simulink model "danhgia_chatluong_chuabutre"  (R2020a)
settings: Solver=ode1be  StartTime=0.0  StopTime=Tmophong  FixedStep=Ts  RelTol=1e-3
values from neighbouring files (symbols this model uses):
  L = 30e-3    (= 0.03)    [init.m]    (also in init_khongbutre.m)
  omega_Ref = 2*pi*50    (= 314.159265359)    [init.m]    (also in init_khongbutre.m)
  R = 6    [init.m]    (also in init_khongbutre.m; kalmanfilter1.m = 4)
  Ts = 50e-6    (= 5e-05)    [init.m]    (also in init_khongbutre.m)
libraries: nesl_utility x18, ee_lib x17, fl_lib x4
settings Model: Creator=tinh  LastModifiedBy=Tinh_deptrai
settings SolverCC: NumberNewtonIterations=3
settings DataIOCC: ExternalInput=sinA,sinB,sinC  LoadExternalInput=on
settings SimscapeCC: SimscapeLogToSDI=on

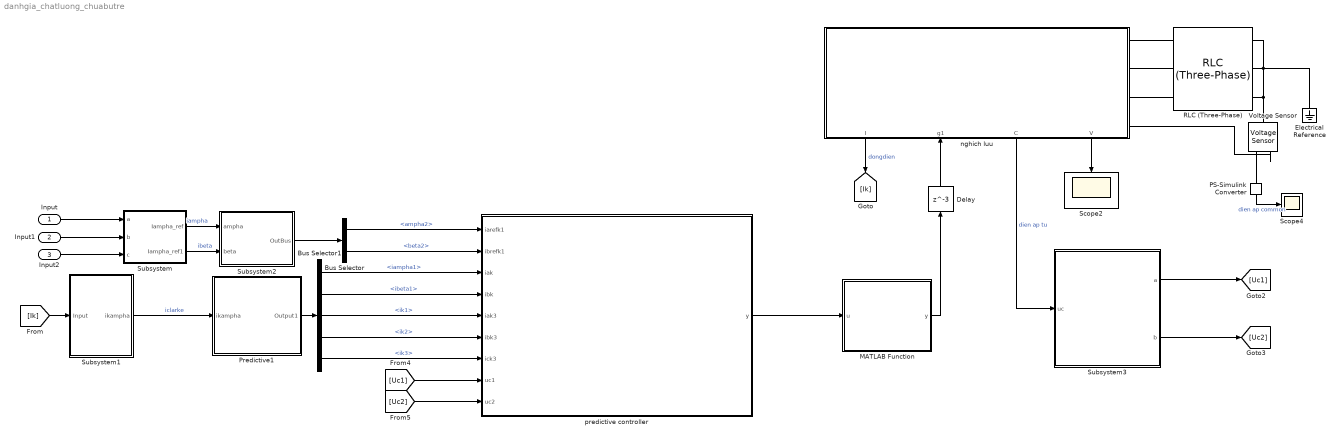
== system danhgia_chatluong_chuabutre ==
  Input : Inport
  Input1 : Inport  Port=2
  Input2 : Inport  Port=3
  Bus Selector : BusSelector  OutputSignals=ampha2,beta2
  Bus Selector1 : BusSelector  OutputSignals=iampha1,ibeta1,ik1,ik2,ik3
  Delay : Delay  DelayLength=3
  Electrical Reference : fl_lib/Electrical/Electrical Elements/Electrical Reference
  MATLAB Function : MATLAB Function  TreatAsAtomicUnit=on
  PS-Simulink Converter : nesl_utility/PS-Simulink Converter  PhysicalDomain=network_engine_domain  SubClassName=ps_output  LeftPortType=input  RightPortType=output  PseudoPeriodic=off  Frequencies=[]  Unit=inherit  AffineConversion=off
  Predictive1 : Subsystem
  RLC (Three-Phase) : ee_lib/Passive/RLC Assemblies/RLC (Three-Phase)  component_structure=4  R=R Ohm  L=L H  IL0=[0, 0, 0] A  C=1e-6 F  VC0=[0, 0, 0] V  R_parasitic=1e-6 Ohm  G_parasitic=1e-6 1/Ohm
      settings: SourceProductBaseCode=PS  InternalSimscapePortConfiguration="{\"Bottom\":[],\"Left\":[{\"id\":\"a1\",\"label\":\"a1\",\"type\":\"foundation.electrical.electrical\"},{\"id\":\"b1\",\"label\":\"b1\",\"type\":\"foundation.electrical.electrical\"},{\"id\":\"c1\",\"label\":\"c1\",\"type\":\"foundation.electrical.electrical\"}],\"Right\":[{\"id\":\"a2\",\"label\":\"a2\",\"type\":\"foundation.electrical.electrical\"},{\"id\":\"b2\",\"label\":\"b2\",\"type\":\"foundation.electrical.electrical\"},{\"id\":\"c2\",\"label\":\"c2\",\"type\":\"foundation.electrical.electrical\"}],\"Top\":[]}"
  Scope2 : Scope
  Scope4 : Scope
  Subsystem : Subsystem
  Subsystem1 : Subsystem
  Subsystem2 : Subsystem
  Subsystem3 : Subsystem
  Voltage Sensor : fl_lib/Electrical/Electrical Sensors/Voltage Sensor
  nghich luu : Subsystem
      settings: PortSchema="{\"entries\":[{\"content\":{\"sides\":[{\"content\":{\"connectorIds\":[]},\"type\":\"ConnectorPlacement.EquallySpacedRectSide\",\"uuid\":\"1f21bf9d-b3c4-4ef8-831a-50a976b6aa65\"},{\"content\":{\"connectorIds\":[\"RConn1\",\"RConn2\",\"RConn3\",\"RConn4\"],\"side\":\"RIGHT\"},\"type\":\"ConnectorPlacement.EquallySpacedRectSide\",\"uuid\":\"0787168a-1f3c-4831-aef7-a1860c607723\"},{\"content\":{\"connectorIds\":[],\"side\":\"TOP\"},\"type\":\"ConnectorPlacement.EquallySpacedRectSide\",\"uuid\":\"c9cfdced-0897-45ca-aa61-726ea781df92\"},{\"content\":{\"connectorIds\":[\"Out1\",\"In1\",\"Out2\",\"Out3\"],\"side\":\"BOTTOM\"},\"type\":\"ConnectorPlacement.EquallySpacedRectSide\",\"uuid\":\"0f797b02-a78f-4846-a0f4-57f75c54f7ea\"}]},\"type\":\"ConnectorPlacement.EquallySpacedConnector\",\"uuid\":\"5e077d9d-cbda-4f20-95e3-2cacb065a3ee\"}],\"packageUris\":[\"http://schema.mathworks.com/mf0/Connector/19700101\"],\"version\":\"1.0\"}"
  predictive controller : MATLAB Function  TreatAsAtomicUnit=on
  wires:
  Input2/1 -> Subsystem/3(c)
  Subsystem/1(Iampha_ref) -> Subsystem2/1(ampha)  "iampha"
  Subsystem/2(Iampha_ref1) -> Subsystem2/2(beta)  "ibeta"
  Input/1 -> Subsystem/1(a)
  Input1/1 -> Subsystem/2(b)
  MATLAB Function/1(y) -> Delay/1
  Delay/1 -> nghich luu/1(g1)
  nghich luu/2(C) -> Subsystem3/1(uc)  "dien ap tu"
  nghich luu/3(V) -> Scope2/1
  nghich luu/1(I) -> [Ik]  "dongdien"
  Bus Selector/1 -> predictive controller/1(iarefk1)  "<ampha2>"
  Bus Selector/2 -> predictive controller/2(ibrefk1)  "<beta2>"
  Subsystem2/1(OutBus) -> Bus Selector/1
  Bus Selector1/1 -> predictive controller/3(iak)  "<iampha1>"
  Bus Selector1/2 -> predictive controller/4(ibk)  "<ibeta1>"
  Bus Selector1/3 -> predictive controller/5(iak3)  "<ik1>"
  Bus Selector1/4 -> predictive controller/6(ibk3)  "<ik2>"
  Bus Selector1/5 -> predictive controller/7(ick3)  "<ik3>"
  Subsystem3/1(a) -> [Uc1]
  Subsystem3/2(b) -> [Uc2]
  PS-Simulink Converter/1 -> Scope4/1  "dien ap common"
  Predictive1/1(Output1) -> Bus Selector1/1
  [Ik] -> Subsystem1/1(Input)
  Subsystem1/1(ikampha) -> Predictive1/1(ikampha)  "iclarke"
  [Uc1] -> predictive controller/8(uc1)
  [Uc2] -> predictive controller/9(uc2)
  predictive controller/1(y) -> MATLAB Function/1(u)
  connections:
  RLC (Three-Phase)/RConn3 -- RLC (Three-Phase)/RConn2 -- RLC (Three-Phase)/RConn1 -- Electrical Reference/LConn1 -- Voltage Sensor/LConn1
  RLC (Three-Phase)/LConn1 -- nghich luu/RConn1
  RLC (Three-Phase)/LConn2 -- nghich luu/RConn2
  RLC (Three-Phase)/LConn3 -- nghich luu/RConn3
  Voltage Sensor/RConn2 -- nghich luu/RConn4
  PS-Simulink Converter/LConn1 -- Voltage Sensor/RConn1

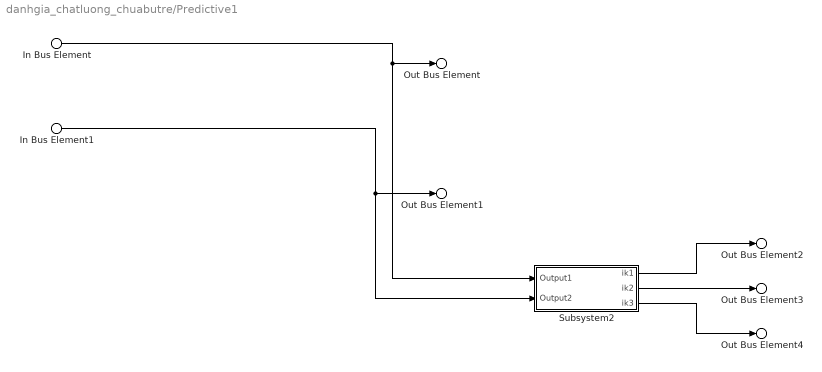
== system danhgia_chatluong_chuabutre/Predictive1 ==
  In Bus Element : Inport  PortName=ikampha  Element=Iampha
  In Bus Element1 : Inport  PortName=ikampha  Element=Ibeta
  Subsystem2 : Subsystem
  Out Bus Element : Outport  PortName=Output1  Element=iampha1
  Out Bus Element1 : Outport  PortName=Output1  Element=ibeta1
  Out Bus Element2 : Outport  PortName=Output1  Element=ik1
  Out Bus Element3 : Outport  PortName=Output1  Element=ik2
  Out Bus Element4 : Outport  PortName=Output1  Element=ik3
  wires:
  In Bus Element/1 -> Out Bus Element/1, Subsystem2/1(Output1)
  In Bus Element1/1 -> Out Bus Element1/1, Subsystem2/2(Output2)
  Subsystem2/1(ik1) -> Out Bus Element2/1
  Subsystem2/2(ik2) -> Out Bus Element3/1
  Subsystem2/3(ik3) -> Out Bus Element4/1

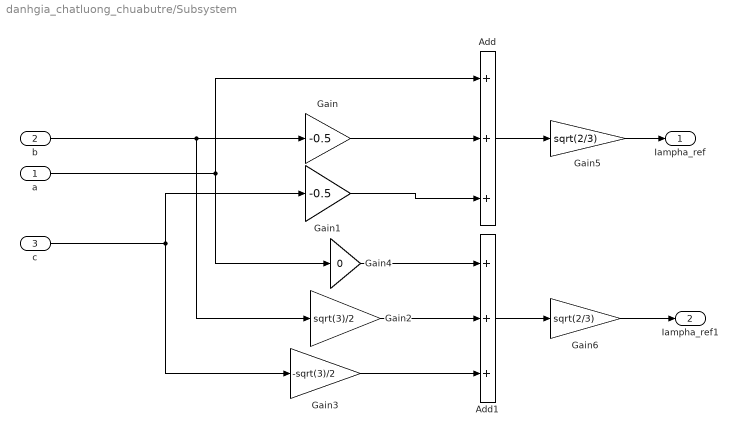
== system danhgia_chatluong_chuabutre/Subsystem ==
  a : Inport
  b : Inport  Port=2
  c : Inport  Port=3
  Add : Sum  Inputs=+++
  Add1 : Sum  Inputs=+++
  Gain : Gain  Gain=-0.5
  Gain1 : Gain  Gain=-0.5
  Gain2 : Gain  Gain=sqrt(3)/2
  Gain3 : Gain  Gain=-sqrt(3)/2
  Gain4 : Gain  Gain=0
  Gain5 : Gain  Gain=sqrt(2/3)
  Gain6 : Gain  Gain=sqrt(2/3)
  Iampha_ref : Outport
  Iampha_ref1 : Outport  Port=2
  wires:
  Add1/1 -> Gain6/1
  Gain3/1 -> Add1/3
  Gain2/1 -> Add1/2
  Gain1/1 -> Add/3
  c/1 -> Gain3/1, Gain1/1
  Gain/1 -> Add/2
  b/1 -> Gain2/1, Gain/1
  Add/1 -> Gain5/1
  a/1 -> Add/1, Gain4/1
  Gain4/1 -> Add1/1
  Gain5/1 -> Iampha_ref/1
  Gain6/1 -> Iampha_ref1/1

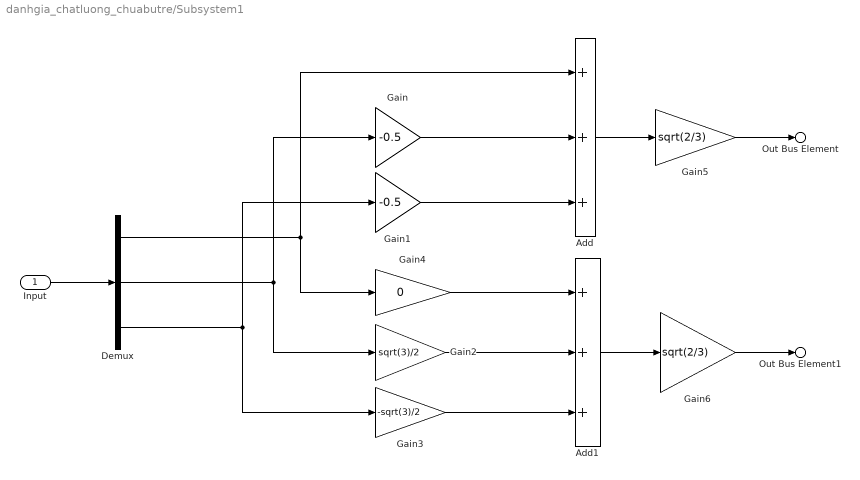
== system danhgia_chatluong_chuabutre/Subsystem1 ==
  Input : Inport
  Add : Sum  Inputs=+++
  Add1 : Sum  Inputs=+++
  Demux : Demux  Outputs=3
  Gain : Gain  Gain=-0.5
  Gain1 : Gain  Gain=-0.5
  Gain2 : Gain  Gain=sqrt(3)/2
  Gain3 : Gain  Gain=-sqrt(3)/2
  Gain4 : Gain  Gain=0
  Gain5 : Gain  Gain=sqrt(2/3)
  Gain6 : Gain  Gain=sqrt(2/3)
  Out Bus Element : Outport  PortName=ikampha  Element=Iampha
  Out Bus Element1 : Outport  PortName=ikampha  Element=Ibeta
  wires:
  Add1/1 -> Gain6/1
  Gain3/1 -> Add1/3
  Gain2/1 -> Add1/2
  Gain1/1 -> Add/3
  Demux/3 -> Gain3/1, Gain1/1
  Gain/1 -> Add/2
  Demux/2 -> Gain2/1, Gain/1
  Add/1 -> Gain5/1
  Demux/1 -> Add/1, Gain4/1
  Gain4/1 -> Add1/1
  Gain5/1 -> Out Bus Element/1
  Gain6/1 -> Out Bus Element1/1
  Input/1 -> Demux/1

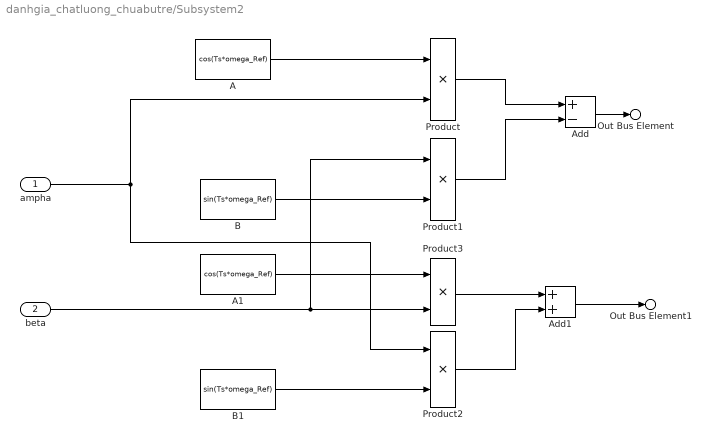
== system danhgia_chatluong_chuabutre/Subsystem2 ==
  ampha : Inport
  beta : Inport  Port=2
  A : Constant  Value=cos(Ts*omega_Ref)
  A1 : Constant  Value=cos(Ts*omega_Ref)
  Add : Sum  Inputs=+-
  Add1 : Sum
  B : Constant  Value=sin(Ts*omega_Ref)
  B1 : Constant  Value=sin(Ts*omega_Ref)
  Product{,1..3} (4 alike) : Product
  Out Bus Element : Outport  PortName=OutBus  Element=ampha2
  Out Bus Element1 : Outport  PortName=OutBus  Element=beta2
  wires:
  A/1 -> Product/1
  B/1 -> Product1/2
  ampha/1 -> Product2/1, Product/2
  beta/1 -> Product1/1, Product3/2
  A1/1 -> Product3/1
  B1/1 -> Product2/2
  Product/1 -> Add/1
  Product1/1 -> Add/2
  Product3/1 -> Add1/1
  Product2/1 -> Add1/2
  Add/1 -> Out Bus Element/1
  Add1/1 -> Out Bus Element1/1

== system danhgia_chatluong_chuabutre/Subsystem3 ==
  uc : Inport
  Demux1 : Demux  Outputs=2
  a : Outport
  b : Outport  Port=2
  wires:
  uc/1 -> Demux1/1
  Demux1/1 -> a/1
  Demux1/2 -> b/1

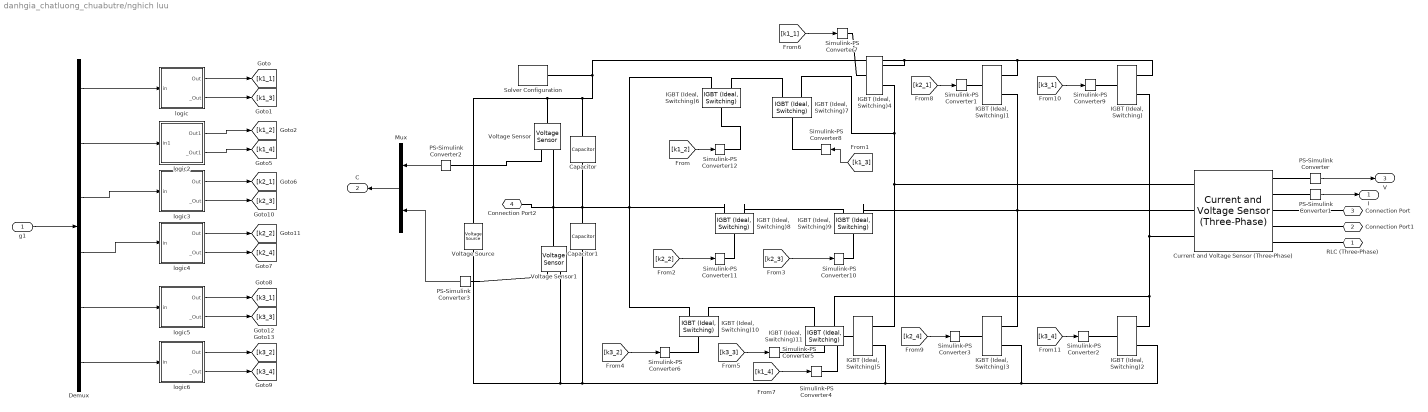
== system danhgia_chatluong_chuabutre/nghich luu ==
  g1 : Inport
  Capacitor : ee_lib/Passive/Capacitor  cap_option=0  c=0.0022 F  Cvec=[1e-05, 1e-06] F  Vvec=[0, 10] V  CV_table_symmetry=1  f_vec=[1, 10] kHz  DFext_vec=[.8, 1.2]  C_tol=5  enable_C_tol=0  tol_distribution=1  nSigma=4  r=1e-6 Ohm  g=0 1/Ohm  averaging_period=0 s  enable_operating_limits=1  operating_limit_action=2  max_working_voltage_range=[30, 60] V  power_rating=200 W  enable_faults=0  fault_action=1  Cscale_faulted=100  R_faulted=1e-3 Ohm  G_faulted=0 1/Ohm  tau_fault=1e-3 s  enable_temporal_fault=0  t_fault=1 s  enable_behavioral_fault=0  max_permissible_voltage_range=[-100, 100] V  t_fail_on_voltage=1 s  i_specify=off  i_priority=None  i=0 A  i_nominal_specify=off  i_nominal_unit=A  i_nominal_value=1  v_specify=on  v_priority=High  v=50 V  v_nominal_specify=off  v_nominal_unit=V  v_nominal_value=1  vc_specify=on  vc_priority=High  vc=50 V  vc_nominal_specify=off  vc_nominal_unit=V  vc_nominal_value=1
  Capacitor1 : ee_lib/Passive/Capacitor  cap_option=0  c=0.0022 F  Cvec=[1e-05, 1e-06] F  Vvec=[0, 10] V  CV_table_symmetry=1  f_vec=[1, 10] kHz  DFext_vec=[.8, 1.2]  C_tol=5  enable_C_tol=0  tol_distribution=1  nSigma=4  r=1e-6 Ohm  g=0 1/Ohm  averaging_period=0 s  enable_operating_limits=1  operating_limit_action=2  max_working_voltage_range=[30, 60] V  power_rating=200 W  enable_faults=0  fault_action=1  Cscale_faulted=100  R_faulted=1e-3 Ohm  G_faulted=0 1/Ohm  tau_fault=1e-3 s  enable_temporal_fault=0  t_fault=1 s  enable_behavioral_fault=0  max_permissible_voltage_range=[-100, 100] V  t_fail_on_voltage=1 s  i_specify=off  i_priority=None  i=0 A  i_nominal_specify=off  i_nominal_unit=A  i_nominal_value=1  v_specify=on  v_priority=High  v=50 V  v_nominal_specify=off  v_nominal_unit=V  v_nominal_value=1  vc_specify=on  vc_priority=High  vc=50 V  vc_nominal_specify=off  vc_nominal_unit=V  vc_nominal_value=1
  Current and Voltage Sensor (Three-Phase) : ee_lib/Sensors & Transducers/Current and Voltage Sensor (Three-Phase)  vMeasurementType=ee.enum.vmeasurement.lg  outputUnit=ee.enum.unit.si  SRated=100e6 V*A  VRated=24e3 V  I_specify=off  I_priority=None  I=[ 0 0 0 ] A  I_nominal_specify=off  I_nominal_unit=A  I_nominal_value=1  V_specify=off  V_priority=None  V=[ 0 0 0 ] V  V_nominal_specify=off  V_nominal_unit=V  V_nominal_value=1
      settings: SourceProductBaseCode=PS  InternalSimscapePortConfiguration="{\"Bottom\":[],\"Left\":[{\"id\":\"a1\",\"label\":\"a1\",\"type\":\"foundation.electrical.electrical\"},{\"id\":\"b1\",\"label\":\"b1\",\"type\":\"foundation.electrical.electrical\"},{\"id\":\"c1\",\"label\":\"c1\",\"type\":\"foundation.electrical.electrical\"}],\"Right\":[{\"id\":\"V_output\",\"label\":\"V\",\"type\":\"output\"},{\"id\":\"I_output\",\"label\":\"I\",\"type\":\"output\"},{\"id\":\"a2\",\"label\":\"a2\",\"type\":\"foundation.electrical.electrical\"},{\"id\":\"b2\",\"label\":\"b2\",\"type\":\"foundation.electrical.electrical\"},{\"id\":\"c2\",\"label\":\"c2\",\"type\":\"foundation.electrical.electrical\"}],\"Top\":[]}"
  Demux : Demux  Outputs=6
  IGBT (Ideal, Switching){,1..11} (12 alike) : ee_lib/Semiconductors & Converters/IGBT (Ideal, Switching)  Vf=0.8 V  Ron=0.001 Ohm  Goff=1e-6 1/Ohm  Vth=0.5 V  diode_param=2  diode_Vf=0.8 V  diode_Ron=0.001 Ohm  diode_Goff=1e-6 1/Ohm  diode_C=50e-9 F  diode_iRM=-235 A  diode_iF=300 A  diode_idot=-50 A/us  diode_trr_param=1  diode_trr_factor=3  diode_trr=15 us  diode_Qrr=1500 s*uA  thermal_loss_option=2  Voff=300 V  Tau=1e-4 s  Tj=[298.15, 398.15] K  Iout_scalar=600 A  Eon_scalar=22.86e-3 J  Eoff_scalar=17.14e-3 J  Von_scalar=2.7 V  Iout_data=[0, 10, 50, 100, 200, 400, 600] A  Eon_data=[0, .29, 1.43, 2.86, 5.71, 13.14, 22.86; 0, .57, 2.63, 5.14, 10.29, 20.57, 30.29] * 1e-3 J  Eoff_data=[0, .21, 1.07, 2.14, 4.29, 9.86, 17.14; 0, .43, 1.97, 3.86, 7.71, 15.43, 22.71] * 1e-3 J  Von_data=[0, 1.1, 1.3, 1.45, 1.75, 2.25, 2.7; 0, 1, 1.15, 1.35, 1.7, 2.35, 3] V
  Mux : Mux  Inputs=2
  PS-Simulink Converter : nesl_utility/PS-Simulink Converter  PhysicalDomain=network_engine_domain  SubClassName=ps_output  LeftPortType=input  RightPortType=output  PseudoPeriodic=off  Frequencies=[]  Unit=inherit  AffineConversion=off
  PS-Simulink Converter1 : nesl_utility/PS-Simulink Converter  PhysicalDomain=network_engine_domain  SubClassName=ps_output  LeftPortType=input  RightPortType=output  PseudoPeriodic=off  Frequencies=[]  Unit=inherit  AffineConversion=off
  PS-Simulink Converter2 : nesl_utility/PS-Simulink Converter  PhysicalDomain=network_engine_domain  SubClassName=ps_output  LeftPortType=input  RightPortType=output  PseudoPeriodic=off  Frequencies=[]  Unit=V  AffineConversion=off
  PS-Simulink Converter3 : nesl_utility/PS-Simulink Converter  PhysicalDomain=network_engine_domain  SubClassName=ps_output  LeftPortType=input  RightPortType=output  PseudoPeriodic=off  Frequencies=[]  Unit=V  AffineConversion=off
  Simulink-PS Converter{1..12} (12 alike) : nesl_utility/Simulink-PS Converter  PhysicalDomain=network_engine_domain  SubClassName=ps_input  LeftPortType=input  RightPortType=output  PseudoPeriodic=off  Frequencies=[]  NoiseDistribution=none  NoiseParameters=[]  Unit=V  AffineConversion=off  FilteringAndDerivatives=provide  SimscapeFilterOrder=1  InputFilterTimeConstant=0.001  UdotUserProvided=0
  Solver Configuration : nesl_utility/Solver Configuration  PhysicalDomain=network_engine_domain  SubClassName=solver  LeftPortType=input  RightPortType=generic  Tones=[]  Harmonics=[]  SimulateNoise=off  Profile=off  UseLocalSampling=off  EnableSwitchedLinearOptims=on  FrequencyDomain=off  UseCCode=off  RelTol=0.001  AbsTol=1e-06  MinStep=1e-09  ToWorkspace=off  RevertToSquareIcSolve=off  NumHomotopyIterations=100  PhasorMode=off  PhasorModeNumHarmonics=1  DoDC=off  ResidualTolerance=10e-06  UseLocalSolver=on  LocalSolverChoice=NE_TRAPEZOIDAL_ADVANCER  LocalSolverSampleTime=Ts  DoFixedCost=off  MaxNonlinIter=3  MaxModeIter=2  LinearAlgebra=auto  EquationFormulation=NE_TIME_EF  DelaysMemoryBudget=1024  AutomaticFiltering=on  FilteringTimeConstant=0.001  PartitionStorageMethod=AS_NEEDED  PartitionMemoryBudget=1024  PartitionMethod=ROBUST
  Voltage Sensor : fl_lib/Electrical/Electrical Sensors/Voltage Sensor
  Voltage Sensor1 : fl_lib/Electrical/Electrical Sensors/Voltage Sensor
  Voltage Source : ee_lib/Sources/Voltage Source  dc_voltage=Vdc V  ac_voltage=0 V  ac_shift=0 rad  ac_frequency=0 Hz  noise_mode=0  PSD=0 V^2/Hz  repeatability=1  auto_seed=418932850  user_seed=0  sample_time=1e-3 s  i_specify=off  i_priority=None  i=0 A  i_nominal_specify=off  i_nominal_unit=A  i_nominal_value=1  v_specify=off  v_priority=None  v=0 V  v_nominal_specify=off  v_nominal_unit=V  v_nominal_value=1
  logic : Subsystem
  logic2 : Subsystem
  logic3 : Subsystem
  logic4 : Subsystem
  logic5 : Subsystem
  logic6 : Subsystem
  RLC (Three-Phase) : PMIOPort  Side=Right
  Connection Port1 : PMIOPort  Port=2  Side=Right
  Connection Port : PMIOPort  Port=3  Side=Right
  Connection Port2 : PMIOPort  Port=4  Side=Right
  I : Outport
  C : Outport  Port=2
  V : Outport  Port=3
  wires:
  [k1_2] -> Simulink-PS Converter12/1
  [k1_3] -> Simulink-PS Converter8/1
  [k2_2] -> Simulink-PS Converter11/1
  [k2_3] -> Simulink-PS Converter10/1
  [k3_2] -> Simulink-PS Converter6/1
  [k3_3] -> Simulink-PS Converter5/1
  [k1_1] -> Simulink-PS Converter7/1
  [k2_1] -> Simulink-PS Converter1/1
  [k3_1] -> Simulink-PS Converter9/1
  [k1_4] -> Simulink-PS Converter4/1
  [k2_4] -> Simulink-PS Converter3/1
  [k3_4] -> Simulink-PS Converter2/1
  PS-Simulink Converter3/1 -> Mux/2
  PS-Simulink Converter2/1 -> Mux/1
  Mux/1 -> C/1
  logic/2(_Out) -> [k1_3]
  Demux/1 -> logic/1(in)
  g1/1 -> Demux/1
  logic/1(Out) -> [k1_1]
  logic2/1(Out1) -> [k1_2]
  logic2/2(_Out1) -> [k1_4]
  logic3/1(Out) -> [k2_1]
  logic3/2(_Out) -> [k2_3]
  logic4/1(Out) -> [k2_2]
  logic4/2(_Out) -> [k2_4]
  logic5/1(Out) -> [k3_1]
  logic5/2(_Out) -> [k3_3]
  logic6/1(Out) -> [k3_2]
  logic6/2(_Out) -> [k3_4]
  Demux/6 -> logic6/1(in)
  Demux/5 -> logic5/1(in)
  Demux/4 -> logic4/1(in)
  Demux/3 -> logic3/1(in)
  Demux/2 -> logic2/1(in1)
  PS-Simulink Converter/1 -> V/1
  PS-Simulink Converter1/1 -> I/1
  connections:
  Voltage Source/LConn1 -- "IGBT (Ideal, Switching)4"/RConn1 -- "IGBT (Ideal, Switching)1"/RConn1 -- "IGBT (Ideal, Switching)"/RConn1 -- Solver Configuration/RConn1 -- Capacitor/LConn1 -- Voltage Sensor/LConn1
  Voltage Source/RConn1 -- Voltage Sensor1/RConn2 -- "IGBT (Ideal, Switching)3"/RConn2 -- "IGBT (Ideal, Switching)2"/RConn2 -- "IGBT (Ideal, Switching)5"/RConn2 -- Capacitor1/RConn1
  Capacitor/RConn1 -- Voltage Sensor/RConn2 -- Connection Port2/RConn1 -- Voltage Sensor1/LConn1 -- "IGBT (Ideal, Switching)6"/RConn1 -- "IGBT (Ideal, Switching)8"/RConn1 -- "IGBT (Ideal, Switching)10"/RConn1 -- Capacitor1/LConn1
  "IGBT (Ideal, Switching)3"/RConn1 -- "IGBT (Ideal, Switching)1"/RConn2 -- "IGBT (Ideal, Switching)9"/RConn1 -- Current and Voltage Sensor (Three-Phase)/LConn2
  "IGBT (Ideal, Switching)7"/RConn2 -- "IGBT (Ideal, Switching)6"/RConn2
  "IGBT (Ideal, Switching)8"/RConn2 -- "IGBT (Ideal, Switching)9"/RConn2
  "IGBT (Ideal, Switching)11"/RConn2 -- "IGBT (Ideal, Switching)10"/RConn2
  "IGBT (Ideal, Switching)4"/RConn2 -- "IGBT (Ideal, Switching)7"/RConn1 -- "IGBT (Ideal, Switching)5"/RConn1 -- Current and Voltage Sensor (Three-Phase)/LConn1
  "IGBT (Ideal, Switching)"/RConn2 -- "IGBT (Ideal, Switching)2"/RConn1 -- "IGBT (Ideal, Switching)11"/RConn1 -- Current and Voltage Sensor (Three-Phase)/LConn3
  Simulink-PS Converter12/RConn1 -- "IGBT (Ideal, Switching)6"/LConn1
  Simulink-PS Converter8/RConn1 -- "IGBT (Ideal, Switching)7"/LConn1
  Simulink-PS Converter10/RConn1 -- "IGBT (Ideal, Switching)9"/LConn1
  Simulink-PS Converter6/RConn1 -- "IGBT (Ideal, Switching)10"/LConn1
  Simulink-PS Converter5/RConn1 -- "IGBT (Ideal, Switching)11"/LConn1
  "IGBT (Ideal, Switching)3"/LConn1 -- Simulink-PS Converter3/RConn1
  "IGBT (Ideal, Switching)2"/LConn1 -- Simulink-PS Converter2/RConn1
  "IGBT (Ideal, Switching)4"/LConn1 -- Simulink-PS Converter7/RConn1
  "IGBT (Ideal, Switching)1"/LConn1 -- Simulink-PS Converter1/RConn1
  "IGBT (Ideal, Switching)"/LConn1 -- Simulink-PS Converter9/RConn1
  "IGBT (Ideal, Switching)5"/LConn1 -- Simulink-PS Converter4/RConn1
  PS-Simulink Converter2/LConn1 -- Voltage Sensor/RConn1
  PS-Simulink Converter3/LConn1 -- Voltage Sensor1/RConn1
  Simulink-PS Converter11/RConn1 -- "IGBT (Ideal, Switching)8"/LConn1
  Connection Port/RConn1 -- Current and Voltage Sensor (Three-Phase)/RConn3
  Connection Port1/RConn1 -- Current and Voltage Sensor (Three-Phase)/RConn4
  RLC (Three-Phase)/RConn1 -- Current and Voltage Sensor (Three-Phase)/RConn5
  PS-Simulink Converter1/LConn1 -- Current and Voltage Sensor (Three-Phase)/RConn2
  PS-Simulink Converter/LConn1 -- Current and Voltage Sensor (Three-Phase)/RConn1

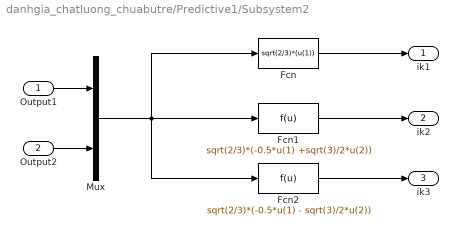
== system danhgia_chatluong_chuabutre/Predictive1/Subsystem2 ==
  Output1 : Inport
  Output2 : Inport  Port=2
  Fcn : Fcn  Expr=sqrt(2/3)*(u(1))
  Fcn1 : Fcn  Expr=sqrt(2/3)*(-0.5*u(1) +sqrt(3)/2*u(2))
  Fcn2 : Fcn  Expr=sqrt(2/3)*(-0.5*u(1) - sqrt(3)/2*u(2))
  Mux : Mux  Inputs=2
  ik1 : Outport
  ik2 : Outport  Port=2
  ik3 : Outport  Port=3
  wires:
  Output1/1 -> Mux/1
  Output2/1 -> Mux/2
  Mux/1 -> Fcn/1, Fcn1/1, Fcn2/1
  Fcn/1 -> ik1/1
  Fcn1/1 -> ik2/1
  Fcn2/1 -> ik3/1

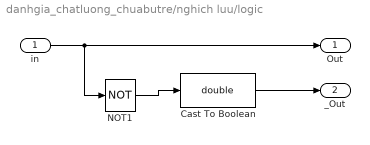
== system danhgia_chatluong_chuabutre/nghich luu/logic ==
  in : Inport
  Cast To Boolean : DataTypeConversion  OutDataTypeStr=double
  NOT1 : Logic  Operator=NOT  IconShape=distinctive  AllPortsSameDT=off  OutDataTypeStr=boolean
  Out : Outport
  _Out : Outport  Port=2
  wires:
  in/1 -> NOT1/1, Out/1
  NOT1/1 -> Cast To Boolean/1
  Cast To Boolean/1 -> _Out/1

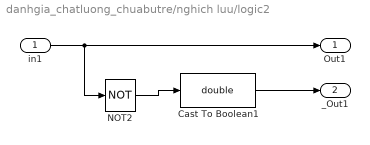
== system danhgia_chatluong_chuabutre/nghich luu/logic2 ==
  in1 : Inport
  Cast To Boolean1 : DataTypeConversion  OutDataTypeStr=double
  NOT2 : Logic  Operator=NOT  IconShape=distinctive  AllPortsSameDT=off  OutDataTypeStr=boolean
  Out1 : Outport
  _Out1 : Outport  Port=2
  wires:
  Cast To Boolean1/1 -> _Out1/1
  in1/1 -> NOT2/1, Out1/1
  NOT2/1 -> Cast To Boolean1/1

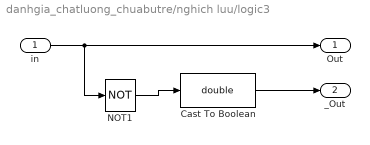
== system danhgia_chatluong_chuabutre/nghich luu/logic3 ==
  in : Inport
  Cast To Boolean : DataTypeConversion  OutDataTypeStr=double
  NOT1 : Logic  Operator=NOT  IconShape=distinctive  AllPortsSameDT=off  OutDataTypeStr=boolean
  Out : Outport
  _Out : Outport  Port=2
  wires:
  Cast To Boolean/1 -> _Out/1
  in/1 -> NOT1/1, Out/1
  NOT1/1 -> Cast To Boolean/1

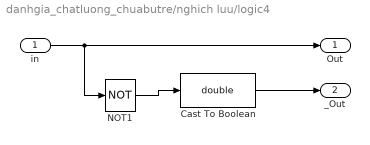
== system danhgia_chatluong_chuabutre/nghich luu/logic4 ==
  in : Inport
  Cast To Boolean : DataTypeConversion  OutDataTypeStr=double
  NOT1 : Logic  Operator=NOT  IconShape=distinctive  AllPortsSameDT=off  OutDataTypeStr=boolean
  Out : Outport
  _Out : Outport  Port=2
  wires:
  Cast To Boolean/1 -> _Out/1
  in/1 -> NOT1/1, Out/1
  NOT1/1 -> Cast To Boolean/1

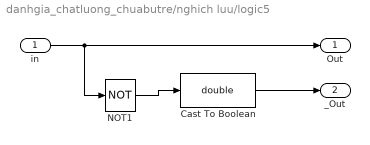
== system danhgia_chatluong_chuabutre/nghich luu/logic5 ==
  in : Inport
  Cast To Boolean : DataTypeConversion  OutDataTypeStr=double
  NOT1 : Logic  Operator=NOT  IconShape=distinctive  AllPortsSameDT=off  OutDataTypeStr=boolean
  Out : Outport
  _Out : Outport  Port=2
  wires:
  Cast To Boolean/1 -> _Out/1
  in/1 -> NOT1/1, Out/1
  NOT1/1 -> Cast To Boolean/1

== system danhgia_chatluong_chuabutre/nghich luu/logic6 ==
  in : Inport
  Cast To Boolean : DataTypeConversion  OutDataTypeStr=double
  NOT1 : Logic  Operator=NOT  IconShape=distinctive  AllPortsSameDT=off  OutDataTypeStr=boolean
  Out : Outport
  _Out : Outport  Port=2
  wires:
  Cast To Boolean/1 -> _Out/1
  in/1 -> NOT1/1, Out/1
  NOT1/1 -> Cast To Boolean/1

== matlab function danhgia_chatluong_chuabutre/MATLAB Function ==
  data: u input; y output
%% Nguyen Trung Tinh 2020
% tinh.nguyenhayho@gmail.com
% tinhhayho@gmail.com
% tin hieu dieu khien cac igbt
% 
%%
function y = fcn(u)
control_signal =...
    [ ...
        0, 1, 0, 1, 0, 1; 0, 0, 0, 0, 0, 0; 1, 1, 1, 1, 1, 1; ...
        1, 1, 0, 1, 0, 1; 0, 1, 0, 0, 0, 0; 1, 1, 1, 1, 0, 1; ...
        0, 1, 0, 1, 0, 0; 0, 1, 1, 1, 0, 1; 0, 0, 0, 1, 0, 0; ...
        0, 1, 1, 1, 1, 1; 0, 0, 0, 1, 0, 1; 0, 1, 0, 1, 1, 1; ...
        0, 0, 0, 0, 0, 1; 1, 1, 0, 1, 1, 1; 0, 1, 0, 0, 0, 1; ...
        1, 1, 0, 0, 0, 0; 1, 1, 0, 1, 0, 0; 1, 1, 1, 1, 0, 0; ...
        0, 1, 1, 1, 0, 0; 0, 0, 1, 1, 0, 0; 0, 0, 1, 1, 0, 1; ...
        0, 0, 1, 1, 1, 1; 0, 0, 0, 1, 1, 1; 0, 0, 0, 0, 1, 1; ...
        0, 1, 0, 0, 1, 1; 1, 1, 0, 0, 1, 1; 1, 1, 0, 0, 0, 1  
    ];
y = (control_signal(u,:))';

== matlab function danhgia_chatluong_chuabutre/predictive controller ==
  data: iarefk1 input; y output; ibrefk1 input; iak input; ibk input; iak3 input; ibk3 input; ick3 input; uc1 input; uc2 input
%% Nguyen Trung Tinh 2020
% tinh.nguyenhayho@gmail.com
% tinhhayho@gmail.com
% ngo vao cua ham ---------
% dong dien du doan k+2   |
% dong dien do duoc k+1   |
% dien ap tu do duoc k+1  |
%-------------------------|
% ngo ra cua bo dieu khien -----------------------|
% trang thai dien ap duoc chon                    |
%-------------------------------------------------|
% parameter --------------------
% R
% L
% Ts

%%
function y = fcn(iarefk1,ibrefk1,iak,ibk,iak3,ibk3,ick3,uc1,uc2)
Vreal =          ...
[0.0        ,  0.0        ,          0.0,...
 0.333333333,  0.333333333,  0.166666667,...
 0.166666667, -0.166666667, -0.166666667,...
-0.333333333, -0.333333333, -0.166666667,...
-0.166666667,  0.166666667,  0.166666667,...
 0.666666667,  0.5        ,  0.333333333,...
 0.0        , -0.333333333, -0.5        ,...
-0.666666667, -0.5        , -0.333333333,...
 0.0        ,  0.333333333,  0.5         
];

Vimag=...
[0.0        ,  0.0        ,         0.0 ,...
 0.0        ,  0.0        ,  0.288675135,...
 0.288675135,  0.288675135,  0.288675135,...
 0.0        ,  0.0        , -0.288675135,...
-0.288675135, -0.288675135, -0.288675135,...
 0.0        ,  0.288675135,  0.577350269,...
 0.577350269,  0.577350269,  0.288675135,...
 0.0        , -0.288675135, -0.577350269,...
-0.577350269, -0.577350269, -0.288675135,...
];
state_p_n= ...    
        [0,0,0,0,0,0 ; 0,1,0,1,0,1 ; 1,0,1,0,1,0 ;...
         1,0,0,0,0,0 ; 0,0,0,1,0,1 ; 1,0,1,0,0,0 ;...
         0,0,0,0,0,1 ; 0,0,1,0,0,0 ; 0,1,0,0,0,1 ;...
         0,0,1,0,1,0 ; 0,1,0,0,0,0 ; 0,0,0,0,1,0 ;...
         0,1,0,1,0,0 ; 1,0,0,0,1,0 ; 0,0,0,1,0,0 ;...
         1,0,0,1,0,1 ; 1,0,0,0,0,1 ; 1,0,1,0,0,1 ;...
         0,0,1,0,0,1 ; 0,1,1,0,0,1 ; 0,1,1,0,0,0 ;...
         0,1,1,0,1,0 ; 0,1,0,0,1,0 ; 0,1,0,1,1,0 ;...
         0,0,0,1,1,0 ; 1,0,0,1,1,0 ; 1,0,0,1,0,0 ...
    ];
% khai bao cho dien ap commom_mode
vcom = ...
    [0,   0,   0  ;-0.5,-0.5,-0.5; 0.5, 0.5, 0.5;...
     0.5, 0,   0  ; 0  ,-0.5,-0.5; 0.5, 0.5, 0  ;...
     0,   0,  -0.5; 0  , 0.5, 0  ;-0.5, 0,  -0.5;...
     0,   0.5, 0.5;-0.5, 0  , 0  ; 0,   0,   0.5;...
    -0.5,-0.5, 0  ; 0.5, 0  , 0.5; 0,  -0.5, 0  ;...
     0.5,-0.5,-0.5; 0.5, 0  ,-0.5; 0.5, 0.5,-0.5;...
     0,   0.5,-0.5;-0.5, 0.5, -0.5  ;-0.5, 0.5, 0  ;...
    -0.5, 0.5, 0.5;-0.5, 0  , 0.5;-0.5,-0.5, 0.5;...
     0,  -0.5, 0.5; 0.5,-0.5, 0.5; 0.5,-0.5, 0  ;...
    ];

Ts = 10e-6;
R = 6;
L = 30e-3;
Vdc = 100;
C = 2200e-6;
g_opt = inf;
x_opt = 0;

    for i=1:27
        iak1 = (1-R*Ts/L)*iak + Ts/L*Vreal(i)*Vdc;
        ibk1 = (1-R*Ts/L)*ibk + Ts/L*Vimag(i)*Vdc;
        uc1k1 = uc1 +Ts/C*(-state_p_n(i,1)*iak3...
                              -state_p_n(i,3)*ibk3...
                              -state_p_n(i,5)*ick3);
                          
        uc2k1 = uc2 +Ts/C*( state_p_n(i,2)*iak3...
                               +state_p_n(i,4)*ibk3...
                               +state_p_n(i,6)*ick3);

        g = abs(iarefk1 - iak1) + abs(ibrefk1 - ibk1) + 0.0*abs(uc1k1 -uc2k1)...
            +0.0*abs(vcom(i,1)+vcom(i,2)+vcom(i,3))/3;
        if ( g < g_opt) 
            g_opt = g;
            x_opt = i;
        end
    end
y = x_opt;
